simulink model "MulticopterModel"  (R2022a)
settings: Solver=ode4  StartTime=0.0  StopTime=inf  FixedStep=0.001  RelTol=1e-3
PreLoadFcn:
  | filepath  = fileparts(get_param(bdroot, 'FileName'));
  | cd(filepath);
InitFcn:
  | Init
values from neighbouring files (symbols this model uses):
  ModelFailEnable = 0    [Init.m]
  ModelInit_RPM = 0    [Init.m]
  ModelParam_BattHoverMinutes = 18    [Init.m]
  ModelParam_BattHoverThr = 0.609    [Init.m]
  ModelParam_envAltitude = -50    [Init.m]
  ModelParam_GlobalNoiseGainSwitch = 0.4    [Init.m]
  ModelParam_GPSEphFinal = 0.3    [Init.m]
  ModelParam_GPSEpvFinal = 0.4    [Init.m]
  ModelParam_GPSFix3DFix = 3    [Init.m]
  ModelParam_GPSSatsVisible = 10    [Init.m]
  ModelParam_motorCr = 842.1    [Init.m]
  ModelParam_motorJm = 0.0001287    [Init.m]
  ModelParam_motorMinThr = 0.05    [Init.m]
  ModelParam_motorT = 0.0214    [Init.m]
  ModelParam_motorWb = 22.83    [Init.m]
  ModelParam_noiseBaroCoupleWithSpeed = 0    [Init.m]
  ModelParam_noiseGPSSampTime = 0.2    [Init.m]
  ModelParam_noisePowerIMU = 0    [Init.m]
  ModelParam_noisePowerOffGainAccel = 0.04    [Init.m]
  ModelParam_noisePowerOffGainAccelZ = 0.03    [Init.m]
  ModelParam_noisePowerOffGainGyro = 0.02    [Init.m]
  ModelParam_noisePowerOffGainGyroZ = 0.025    [Init.m]
  ModelParam_noisePowerOffGainMag = 0.02    [Init.m]
  ModelParam_noisePowerOffGainMagZ = 0.035    [Init.m]
  ModelParam_noisePowerOnGainAccel = 0.8    [Init.m]
  ModelParam_noisePowerOnGainAccelZ = 4.5    [Init.m]
  ModelParam_noisePowerOnGainGyro = 2    [Init.m]
  ModelParam_noisePowerOnGainGyroZ = 1    [Init.m]
  ModelParam_noisePowerOnGainMag = 0.025    [Init.m]
  ModelParam_noisePowerOnGainMagZ = 0.05    [Init.m]
  ModelParam_noiseSampleTimeAccel = 0.001    [Init.m]
  ModelParam_noiseSampleTimeGyro = 0.001    [Init.m]
  ModelParam_noiseSampleTimeMag = 0.01    [Init.m]
  ModelParam_noiseUpperGPS = 0.5    [Init.m]
  ModelParam_noiseUpperWindBodyRatio = 0    [Init.m]
  ModelParam_noiseWindSampTime = 0.001    [Init.m]
  ModelParam_rotorCm = 2.783e-07    [Init.m]
  ModelParam_rotorCt = 1.681e-05    [Init.m]
  ModelParam_uavCCm = [0.0035 0.0039 0.0034]    [Init.m]
  ModelParam_uavCd = 0.055    [Init.m]
  ModelParam_uavDearo = 0.12    [Init.m]
  ModelParam_uavJ = [ModelParam_uavJxx,0,0;0,ModelParam_uavJyy,0;0,0,ModelParam_uavJzz]    [Init.m]
  ModelParam_uavMass = 1.515    [Init.m]
  ModelParam_uavMotNumbs = int8(4)    [Init.m]
  ModelParam_uavR = 0.225    [Init.m]
  ModelParam_uavType = int8(3)    [Init.m]
undefined symbols (not defined in the file or in its folder): d_i, Earth, h_i, ModelParam_GPSEpvInitial, ModelParam_GPSEpvTimeConstant, ModelParam_noiseLowPassFilterCoeAccel, ModelParam_noiseLowPassFilterCoeGyro, ModelParam_timeSamp, Newton, Raphson, WGS84
libraries: simulink x12, aerolibtransform2 x3, sharedtransform x3, aerolibasang x3, aerolibatmos2 x2, aerolibutil x2, shared6dof x1, aerolibconvert2 x1, aerolibobsolete x1, MulticopterModelLib x1, aerolibnav x1, aerolibgravity2 x1
(part 3 of 3)

== matlab function MulticopterModel/Force and Moment Model/Propeller Model/Multicopter/uavTypeDefine ==
  data: uavType input; n_p output; motorPhiVector output; motorThetaVector output; motorPsiVector output; motorRotateDirectionVector output
function [n_p,motorPhiVector,motorThetaVector,motorPsiVector,motorRotateDirectionVector]  = fcn(uavType)
% -1: anticlockwise, 1: clockwise 
TypeMotorDirMatrix=[...
    [-1 -1 -1 0 0 0 0 0];... % Tri 3*1 X           Type1
    [1 1 1 0 0 0 0 0];...    % Tri 3*1 +            Type2
    [-1 -1 1 1 0 0 0 0];... % Quad 4*1 X        Type3
    [-1 -1 1 1 0 0 0 0];... % Quad 4*1 +        Type4
    [1 -1 1 -1 -1 1 0 0];... % Hex 6*1 X         Type5
    [1 -1 1 -1 -1 1 0 0];... % Hex 6*1 +         Type6
    [1 -1 1 -1 1 -1 0 0];... % HexCoa 3*2      Type7
    [1 1 -1 -1 -1 -1 1 1];... % Oct 8*1 X        Type8
    [1 1 -1 -1 -1 -1 1 1];... % Oct 8*1 +        Type9
    [1 -1 1 -1 1 -1 1 -1];... % OctCoa 4*2 X  Type10
    [-1 -1 1 1 0 0 0 0];... % Intel Aero          Type11
    [-1 -1 1 1 0 0 0 0];... % custom              Type12
];

TypeMotorPsiAngMatrix=[...
    [pi/3 pi -pi/3 0 0 0 0 0];...%Type1
    [pi/3 pi -pi/3 0 0 0 0 0];...%Type2
    [pi/4   pi/4+pi     pi/4+3*pi/2     pi/4+pi/2   0 0 0 0];...%Type3
    [pi/2 3*pi/2 0 pi 0 0 0 0];...%Type4
    [pi/2 3/2*pi 3/2*pi+pi/3 pi/2+pi/3 pi/2-pi/3 3/2*pi-pi/3 0 0];...%Type5
    [0 pi pi+pi/3 pi/3 -pi/3 pi-pi/3 0 0];...%Type6
    [pi/3 pi/3 pi pi -pi/3 -pi/3 0 0];...%Type7
    [pi/8 pi+pi/8 pi/8+pi/4 pi-pi/8 -pi/8 3/2*pi-pi/8 3/2*pi+pi/8 pi/2+pi/8];...%Type8
    [0 pi pi/4 3/4*pi -pi/4 pi+pi/4 3/2*pi pi/2];...%Type9
    [pi/4 -pi/4 pi+pi/4 pi-pi/4 -pi/4 pi/4 pi-pi/4 pi+pi/4];...%Type10
    [43*pi/180     223*pi/180      317*pi/180      137*pi/180     0 0 0 0];...%Type11  Intel Aero
    [pi/4   pi/4+pi     pi/4+3*pi/2     pi/4+pi/2   0 0 0 0];...%Type12  custom
];

TypeMotorThetaAngMatrix=[...
    [0 0 0 0 0 0 0 0];...%Type1
    [0 0 0 0 0 0 0 0];...%Type2
    [0 0 0 0 0 0 0 0];...%Type3
    [0 0 0 0 0 0 0 0];...%Type4
    [0 0 0 0 0 0 0 0];...%Type5
    [0 0 0 0 0 0 0 0];...%Type6
    [0 0 0 0 0 0 0 0];...%Type7
    [0 0 0 0 0 0 0 0];...%Type8
    [0 0 0 0 0 0 0 0];...%Type9
    [0 0 0 0 0 0 0 0];...%Type10
    [0 0 0 0 0 0 0 0];...%Type11
    [pi/4   pi/4    pi/4    pi/4    0 0 0 0];...%Type12
    ];
TypeMotorPhiAngMatrix=[...
    [0 0 0 0 0 0 0 0];...%Type1
    [0 0 0 0 0 0 0 0];...%Type2
    [0 0 0 0 0 0 0 0];...%Type3
    [0 0 0 0 0 0 0 0];...%Type4
    [0 0 0 0 0 0 0 0];...%Type5
    [0 0 0 0 0 0 0 0];...%Type6
    [0 0 0 0 0 0 0 0];...%Type7
    [0 0 0 0 0 0 0 0];...%Type8
    [0 0 0 0 0 0 0 0];...%Type9
    [0 0 0 0 0 0 0 0];...%Type10
    [0 0 0 0 0 0 0 0];...%Type11
    [0 0 0 0 0 0 0 0];...%Type12
];

TypeMotorNonVector=int8([3;3;4;4;6;6;6;8;8;8;4;4]);

if uavType<0||uavType>length(TypeMotorNonVector)
    uavType=int8(1);
end

motorRotateDirectionVector=TypeMotorDirMatrix(uavType,:);
motorPsiVector=TypeMotorPsiAngMatrix(uavType,:);
motorThetaVector=TypeMotorThetaAngMatrix(uavType,:);
motorPhiVector=TypeMotorPhiAngMatrix(uavType,:);
n_p = TypeMotorNonVector(uavType);

== matlab function MulticopterModel/Force and Moment Model/Propeller Model/Car/MATLAB Function ==
  data: Fb output; Mb output; MotorRads input
function [Fb,Mb] = fcn(MotorRads)

Mb = [0;0;0];
Fb = [0;0;0];

Fb(1)=MotorRads(1)+MotorRads(3);
Mb(3)=MotorRads(1)*0.1-MotorRads(3)*0.1;

== matlab function MulticopterModel/OutputPort1/HILGPSModel/GenCogVel ==
  data: v output; u input; cot output
function [v,cot] = Ang360(u)
v=norm(u(1:2));

if v < 1
    cot = 0;
else
    cot=atan2d(u(2),u(1));
end
 
if cot<0
    cot=cot+360;
end

== matlab function MulticopterModel/Force and Moment Model/Body AeroCenter ==
  data: Fd output; Md output; wb input; Vb input; Cd input; CCm input; uavDearo input
function [Fd,Md] = fcn(wb,Vb,Cd, CCm, uavDearo)
% This is control effectiveness model, where Fb is the force produced by motors, Mb is
% the moment produced by motors, and Fd is the resistance produced by the air.
% The gyroscopic torque is not considered here.
% uavDearo 机身重心位置，向下为正

 Fd = -Cd*Vb.*abs(Vb);%
 
 Mfd=[Fd(2)*uavDearo;-Fd(1)*uavDearo;0];
 
Md=-CCm.*wb.*abs(wb);
Md=Mfd+Md;
%  CCm=4.72e-3;
%  Md=-CCm*wb.*abs(wb)*0.5;%0.3
%  Md= Mfd+Md;
 
end

== matlab function MulticopterModel/OutputPort1/Model Fail Assessment ==
  settings: updateMethod=DISCRETE
  data: ModelFailEnable input; landed input; FailInfo output; ve input; xe input; wb input; ang input
function FailInfo  = fcn(ModelFailEnable,landed,ve,xe,wb,ang)

persistent xTemp;
if isempty(xTemp)
     xTemp=zeros(8,1);
end

persistent kk;
if isempty(kk)
     kk=0;
end

persistent ss;
if isempty(ss)
     ss=zeros(6,1);
end

if ~ModelFailEnable&&(kk<0.5)
    xTemp=zeros(8,1);
    kk=0;
    ss=[xe;ang];
end

if ModelFailEnable&&~landed
    xTemp(1:4,1)=[norm(xe-ss(1:3,1));norm(ve);norm(ang-ss(4:6,1));norm(wb)];
    xTemp(5:8,1)= (xTemp(5:8,1)*kk+xTemp(1:4,1))/(kk+1);
    
    kk=kk+1;
end
%landed = int8(0);
 
FailInfo=xTemp;

== matlab function MulticopterModel/OutputPort1/ZLimit ==
  data: zt input; xe input; Xee output
function Xee = fcn(zt,xe)
Xee=xe;
if Xee(3)>zt
    Xee(3)=zt;
end

== matlab function MulticopterModel/CollisionDetection ==
  settings: updateMethod=DISCRETE
  data: fm output; uFloats input; DCM input; ve input; mass input; t input; tz output; isCrash output
function [fm,tz,isCrash] = fcn(uFloats,DCM,ve,mass,t)

% vect=[1;1;1;1;1;1;1;1];
%是否碰撞标志位
persistent isCol;
if isempty(isCol)
    isCol=int8(0);
end

%输出力和力矩暂存向量
persistent fOut;
if isempty(fOut)
    fOut=[0;0;0;0;0;0];
end    

%碰撞冲量矩阵
persistent mv0;
if isempty(mv0)
    mv0=[0;0;0];
end    

%碰撞时间
persistent tColi;
if isempty(tColi)
    tColi=0;
end      

%如果没有发送碰撞
if isCol<0.5
    %如果收到碰撞消息，且被碰撞物体为编号飞机（带CopterID的值大于0）
    if abs(uFloats(1)-12345)<1 && uFloats(2)>0.5 %如果收到碰撞消息，12345是数据校验位，uFloats(2)是碰撞到飞机的ID
        isCol=int8(1);%设置为碰撞模式
        %被碰撞物体是活动的还是固定的
        if uFloats(3)>0 %被碰撞物与本物体的质量比有正值，说明碰撞物也是飞机，需要用冲量定理
            massOb=mass*uFloats(3)^2;
            veOb = uFloats(7:9); 
            veNew=(mass*ve+massOb*veOb)/(mass+massOb);
        else %被碰撞物为树、房子等固定物体，质量无穷大，直接反弹回去（1/10的速度）
            veNew=-ve/10.0;
        end

        mv0=mass*(veNew-ve);
        tColi=t;%记录碰撞时间
    end        
end

%如果已经发生碰撞
if isCol>=0.5
    if (t-tColi)>0.05
        fOut=[0;0;0;0;0;0];
    else
        %用瞬时的作用力模拟冲量作用（0.05s）
        mv=DCM*mv0;
        mv(1)=mv(1)*(0.7+0.3*rand());
        mv(2)=mv(2)*(0.7+0.3*rand());
        mv(3)=mv(3)*(0.7+0.3*rand());
        fOut(1:3) = mv/0.05;    %冲量除以时间得到力
        fOut(4:6) = rand(3,1)*mass;
    end  
end

%下面处理飞机与场景固定物体之间的碰撞
fm = fOut;
%tz分别表示距地面高度和飞机XYZ坐标
tz=[100;0;0;0];
ddm=[0;0;0;0;0;0];  
if abs(uFloats(1)-12345)<1 %如果收到碰撞消息
    kRa=40;
    kRaVe=5;
    if uFloats(2)<0.5 %如果碰撞的是场景固定物体
        %向下照射射线返回长度
        tz(1)=uFloats(15);
        %飞机在UE4中的坐标
        tz(2:4)=uFloats(4:6);
    else        
        kRa=20;
    end  
    %前后左右是以地面坐标系的北东地为准
    %前障碍物碰撞反馈力
    if uFloats(10)<0 %距前墙面距离，小于0说明已经接触
        z=uFloats(10);
        if z>-0.01
            ddm(1)=-10*ve(1); 
        elseif z>-0.04
            ddm(1)=200*z-20*ve(1); 
        else
            ddm(1)=500*z-50*ve(1); 
        end   
    end
    %后障碍物碰撞反馈力
    if uFloats(11)<0
%         ddm(1)=-uFloats(11)*mass*kRa;
%         if ve(1)<0
%             ddm(1)=ddm(1)-ve(1)*mass*kRaVe;
%         end
        z=uFloats(11);
        if z>-0.01
            ddm(1)=-10*ve(1); 
        elseif z>-0.04
            ddm(1)=-200*z-20*ve(1); 
        else
            ddm(1)=-500*z-50*ve(1); 
        end  

    end 
    %左障碍物碰撞反馈力
    if uFloats(12)<0
%         ddm(2)=-uFloats(12)*mass*kRa;
%         if ve(2)<0
%             ddm(2)=ddm(2)-ve(2)*mass*kRaVe;
%         end
        z=uFloats(12);
        if z>-0.01
            ddm(2)=-10*ve(2); 
        elseif z>-0.04
            ddm(2)=-200*z-20*ve(2); 
        else
            ddm(2)=-500*z-50*ve(2); 
        end 
    end 
    %右障碍物碰撞反馈力
    if uFloats(13)<0
%         ddm(2)=uFloats(13)*mass*kRa;
%         if ve(2)>0
%             ddm(2)=ddm(2)-ve(2)*mass*kRaVe;
%         end
        z=uFloats(13);
        if z>-0.01
            ddm(2)=-10*ve(2); 
        elseif z>-0.04
            ddm(2)=200*z-20*ve(2); 
        else
            ddm(2)=500*z-50*ve(2); 
        end 

    end 
    %上障碍物碰撞反馈力
    if uFloats(14)<0
%         ddm(3)=-uFloats(14)*mass*kRa;
%         if ve(3)<0
%             ddm(3)=ddm(3)-ve(3)*mass*kRaVe;
%         end

        z=uFloats(14);
        if z>-0.01
            ddm(3)=-10*ve(3); 
        elseif z>-0.04
            ddm(3)=-200*z-20*ve(3); 
        else
            ddm(3)=-500*z-50*ve(3); 
        end 
    end
end
%力从地面坐标系映射机体坐标系
ddmm=DCM*ddm(1:3);
fm=fm+[ddmm;0;0;0];

isCrash=isCol;

== matlab function MulticopterModel/OutputPort1/HILGPSModel/MATLAB Function ==
  data: eph input; FixType output
function FixType = fcn(eph)
if eph <= 2
    FixType=3;
elseif eph <= 4
    FixType=2;
else
    FixType=0;
end

== matlab function MulticopterModel/MATLAB Function ==
  settings: updateMethod=DISCRETE
  data: TerrainZ input; y output; tz input
function y = fcn(TerrainZ, tz)
y=TerrainZ;
if tz(1)<=99
    y=tz(4)+tz(1);
end

% persistent last;
% if isempty(last)
%     last=TerrainZ;
% end
% y=TerrainZ;
% if tz(1)<10
%     if tz(1)<0
%         y=last;
%     else
%         y=tz(3)+tz(1);
%     end 
% end

== matlab function MulticopterModel/Crash_Motor_Fault ==
  settings: updateMethod=DISCRETE
  data: u input; y output; isCrash input
function y = fcn(u,isCrash)
y = u;



%如果飞机相撞则损坏三个电机
if isCrash>0.5
    y(1)=rand()/2.0;
    y(2)=rand()/5.0;
    y(3)=rand()/10.0+u(3)*0.9;
end

== matlab function MulticopterModel/Fail Model/Model Failure ==
  settings: updateMethod=DISCRETE
  data: T input; uavMass input; uavR input; isLoadFall input; uavlostMass output; uavlostJ output; LoadFallParams input; isLoadShift input; LoadShiftParams input; isLoadLeak input; LoadLeakParams input; dcm input; deltaM output
function [uavlostMass,uavlostJ,deltaM] = fcn(T,uavMass,uavR,isLoadFall,LoadFallParams,isLoadShift,LoadShiftParams,isLoadLeak,LoadLeakParams,dcm)
% This function aims to calculate the variation of mass and moment of
% inertia caused by model failure including LoadFall, LoadShift, and
% LoadLeak.

persistent tOld;
if isempty(tOld)  
   tOld=0;
end    

deltaM=[0;0;0];

if isLoadFall
    if LoadFallParams(1)>0.95
        LoadFallParams(1)=0.95;
    elseif LoadFallParams(1)<0
        LoadFallParams(1)=0;
    end
    uavlostMass=LoadFallParams(1)*uavMass;
    uavlostJ=zeros(3,3);
elseif isLoadShift
    if LoadShiftParams(1)>0.95
        LoadShiftParams(1)=0.95;
    elseif LoadShiftParams(1)<0
        LoadShiftParams(1)=0;
    end
    
    uavlostMass= 0;
    loadMoveMass= LoadShiftParams(1)*uavMass;
    
    X=uavR*LoadShiftParams(2);
    Y=uavR*LoadShiftParams(3);
    Z=uavR*LoadShiftParams(4);
    
    uavlostJxx= loadMoveMass*(Y^2+Z^2);
    uavlostJyy= loadMoveMass*(X^2+Z^2);
    uavlostJzz= loadMoveMass*(X^2+Y^2);
    uavlostJyz= loadMoveMass*Y*Z;
    uavlostJzx= loadMoveMass*Z*X;
    uavlostJxy= loadMoveMass*X*Y;
    uavlostJ=-[uavlostJxx,-uavlostJxy,-uavlostJzx;-uavlostJxy,uavlostJyy,-uavlostJyz;-uavlostJzx,-uavlostJyz,uavlostJzz];
    
    deltaF = dcm*loadMoveMass*[0;0;9.8];
    
    deltaM = cross([X;Y;Z],deltaF);     % 变化的力矩
    
elseif isLoadLeak
    uavlostJ=zeros(3,3);
    if LoadLeakParams(1)>0.99
        LoadLeakParams(1)=0.99;
    elseif LoadLeakParams(1)<0
        LoadLeakParams(1)=0;
    end
    loadmass0=LoadLeakParams(1)*uavMass;
    
    if tOld<0.01
        tOld=T;
    end
    
    dt=T-tOld;
    
    LoadLeakRatio = LoadLeakParams(2)*dt;
    if LoadLeakRatio > 0.99
        LoadLeakRatio = 0.99;
    end
    uavlostMass = LoadLeakRatio*loadmass0;
    
else
    uavlostMass=0;
    uavlostJ=zeros(3,3);
    tOld=0;
end

if ~isLoadLeak    %reset
    tOld=0;
end

== matlab function MulticopterModel/Force and Moment Model/Propeller Model old Version ==
  data: uavType input; MotorRads input; R input; uavDearo input; Fb output; Mb output; Cm input; Ct input; Jm input; wb input; Vb input; Cd input
function [Fb,Mb] = fcn(uavType,MotorRads,R,uavDearo,Cm,Ct,Jm,wb,Vb,Cd)
% This is control effectiveness model, where Fb is the force produced by motors, Mb is
% the moment produced by motors, and Fd is the resistance produced by the air.
% The gyroscopic torque is not considered here.

% -1: anticlockwise, 1: clockwise 
TypeMotorDirMatrix=[...
    [-1 -1 -1 0 0 0 0 0];... % Tri 3*1 X
    [1 1 1 0 0 0 0 0];...    % Tri 3*1 +
    [-1 -1 1 1 0 0 0 0];... % Quad 4*1 X
    [-1 -1 1 1 0 0 0 0];... % Quad 4*1 +
    [1 -1 1 -1 -1 1 0 0];... % Hex 6*1 X
    [1 -1 1 -1 -1 1 0 0];... % Hex 6*1 +
    [1 -1 1 -1 1 -1 0 0];... % HexCoa 3*2
    [1 1 -1 -1 -1 -1 1 1];... % Oct 8*1 X
    [1 1 -1 -1 -1 -1 1 1];... % Oct 8*1 +
    [1 -1 1 -1 1 -1 1 -1];... % OctCoa 4*2 X
];

TypeMotorAngMatrix=[...
    [pi/3 pi -pi/3 0 0 0 0 0];...
    [pi/3 pi -pi/3 0 0 0 0 0];...
    [pi/4 pi/4+pi pi/4+3*pi/2 pi/4+pi/2 0 0 0 0];...
    [pi/2 3*pi/2 0 pi 0 0 0 0];...
    [pi/2 3/2*pi 3/2*pi+pi/3 pi/2+pi/3 pi/2-pi/3 3/2*pi-pi/3 0 0];...
    [0 pi pi+pi/3 pi/3 -pi/3 pi-pi/3 0 0];...
    [pi/3 pi/3 pi pi -pi/3 -pi/3 0 0];...
    [pi/8 pi+pi/8 pi/8+pi/4 pi-pi/8 -pi/8 3/2*pi-pi/8 3/2*pi+pi/8 pi/2+pi/8];...
    [0 pi pi/4 3/4*pi -pi/4 pi+pi/4 3/2*pi pi/2];...
    [pi/4 -pi/4 pi+pi/4 pi-pi/4 -pi/4 pi/4 pi-pi/4 pi+pi/4];...
];

TypeMotorNonVector=int8([3;3;4;4;6;6;6;8;8;8]);

Mb = [0;0;0];
Fb = [0;0;0];
P=wb(1);Q=wb(2);

if uavType==50
    
    Fb(1)=MotorRads(1)+MotorRads(3);
    Mb(3)=MotorRads(1)*0.1-MotorRads(3)*0.1;
    
    return;
end


if uavType<0||uavType>length(TypeMotorNonVector)
    uavType=int8(1);
end

TypeMotorDirVector=TypeMotorDirMatrix(uavType,:);
TypeMotorAngVector=TypeMotorAngMatrix(uavType,:);

for i=1:TypeMotorNonVector(uavType)
    propAng = TypeMotorAngVector(i);
    propdir = TypeMotorDirVector(i);
    PropT = Ct*MotorRads(i)*MotorRads(i);
    PropM = Cm*MotorRads(i)*MotorRads(i);
    
    %Thrust -> Moment
    Mb=Mb+[-R*sin(propAng)*PropT;R*cos(propAng)*PropT;-PropM*propdir];
    
    %gyroscopic moment
    Mb=Mb+[Q*Jm*MotorRads(i)*propdir;-P*Jm*MotorRads(i)*propdir;0];
    
    Fb=Fb+[0;0;-PropT];
end

 
end

== matlab function MulticopterModel/Force and Moment Model/Ground Model ==
  settings: updateMethod=DISCRETE
  data: mg input; wb input; Xe input; F1 output; Ve input; M1 output; Quet input; terrainZ input; landed output; takeoff output
function [F1,M1,landed,takeoff] = fcn(mg,wb,Xe,Ve,Quet,terrainZ)
% This is a ground model that can provides reaction force and reaction torque

% persistent z0;
% if isempty(z0)
%      z0=0;
% end

persistent takeoffFlag;
if isempty(takeoffFlag)
     takeoffFlag=int8(0);
end

persistent landFlag;
if isempty(landFlag)
     landFlag=int8(1);
end

z=Xe(3)-terrainZ;

if (z<-0.3)&&(Ve(3)<-0.1)&&(takeoffFlag<0.5)
    takeoffFlag=int8(1);
    landFlag=int8(0);
end

if (z>-0.05)&&(Ve(3)>0.1)&&(landFlag<0.5)
    landFlag=int8(1);
    takeoffFlag=int8(0);
end

takeoff = takeoffFlag;
landed = landFlag;


F1=[0;0;0];
M1=[0;0;0];

if z>=0
%     if z>=0.3
%         if Ve(3)>=5
%             F1(3)=-mg(3)-1000*Ve(3);
%         else
%             F1(3)=-mg(3)-500*z-100*Ve(3);  
%         end
%     elseif z>=0.1
%         if Ve(3)>=2
%             F1(3)=-mg(3)-100*Ve(3);
%         else
%             F1(3)=-mg(3)-50*z-100*Ve(3);  
%         end
%     else
%          if Ve(3)>=1
%             F1(3)=-mg(3)-50*Ve(3);
%         else
%             F1(3)=-mg(3)-5*z-50*Ve(3);  
%         end       
%     end
    if z<0.05
        F1(3)=-mg(3)-10*Ve(3); 
    elseif z<0.1
        F1(3)=-mg(3)-0.5*z-20*Ve(3); 
    else
        F1(3)=-mg(3)-1*z-50*Ve(3); 
    end

    F1(1)=-50*Ve(1);
    F1(2)=-50*Ve(2);
    
%     if ~(isnan(Quet(2))||isnan(Quet(3))||isnan(Quet(4)))
%         M1=-200*[Quet(2);Quet(3);Quet(4)]-10*wb;
%     end
    
    M1=-20*[Quet(2);Quet(3);Quet(4)]-5*wb;
    M1 = M1 * abs(mg(3))*0.0333;
end

== matlab function MulticopterModel/Battery Model/MATLAB Function ==
  data: load input; time input; EffRatio output; hover_time input; hover_thr input; motorNumbs input; cell_voltage output; isUseCustomHovTime input; CustomHovTime input; isPowOff input; isLowVoltage input; remainVoltageRatio input; islowCapacity input; remainCapacityRatio input; remCapacity output
function [EffRatio, cell_voltage,remCapacity]= LiPo(load,time,hover_time,hover_thr,motorNumbs,isUseCustomHovTime,CustomHovTime,isPowOff,isLowVoltage,remainVoltageRatio,islowCapacity,remainCapacityRatio)
%% battery model
%================================Constants=================================

delta_t = 0.01;
%max_current = 5.500;                % maximum current per motor             (A)
%aux_current = 0.100;                % current of auxillary components       (A)        
%capacity = 1.000;                   % LiPo current capacity                 (Ah)                                 
%cells = 2;                          % LiPo cell count

%==========================================================================

persistent discharge;
if isempty(discharge)
    discharge = 0;
end

persistent startTime;
if isempty(startTime)
    startTime = 0;
end

persistent reset;
if isempty(reset)
    reset = 0;
end

discharge_capacity=0;

% 低电量故障
if islowCapacity
   hover_time = hover_time*remainCapacityRatio(1);
   isUseCustomHovTime=false;
end


if ~isUseCustomHovTime 
    capacity=1;
    
    if hover_time<0.01
        hover_time=0.01;
    end
    
    hover_current=1/(hover_time*1.4/60);
    current=0;
    for i=1:motorNumbs
        current=current+hover_current*(load(i)/hover_thr)^2;
    end
    aux_current=0.5;
    %current = sum(hover_current .* (load/hover_thr).^2) + aux_current;
    current =(current+aux_current)/double(motorNumbs);
    discharge = current * (delta_t / 3600) + discharge;
    discharge_capacity = discharge / capacity;    
end




%如果启用电池模型且使用自定义续航时间
if isUseCustomHovTime
      hover_time=CustomHovTime*1.4*60;
      if reset<0.5
         startTime=time;
         reset=1;
      end
      if hover_time<0.01
          hover_time=0.01;
      end
     discharge_capacity=(time-startTime)/hover_time;
else
    %使用默认的续航算法
    reset=0;
end


if discharge_capacity<0
    discharge_capacity=0;
end
if discharge_capacity>1
    discharge_capacity=1;
end


%电量与电压的曲线
if (0 <= discharge_capacity) && (discharge_capacity <=0.20)
    cell_voltage = -14.029*discharge_capacity^3 + 16.975*discharge_capacity^2 - 5.3339*discharge_capacity + 4.2;
elseif (0.20 < discharge_capacity) && (discharge_capacity < 0.70)
    cell_voltage = -0.2*discharge_capacity + 3.74;
else
    cell_voltage = -48*discharge_capacity^3 + 89.6*discharge_capacity^2 - 55.08*discharge_capacity + 14.716;
end

if cell_voltage < 0.5
    cell_voltage = 0;
end

% 电池失效故障
if isPowOff
     cell_voltage = 0; 
end

% 低电压故障
if isLowVoltage
    if remainVoltageRatio(1)>1
        remainVoltageRatio(1)=1;
    elseif remainVoltageRatio(1)<0
        remainVoltageRatio(1)=0;
    end
     cell_voltage = remainVoltageRatio(1)*4.2;
end


%如果电池模型未启用，续航为无穷久，同时各个全局变量归零
if ~isUseCustomHovTime&&~isPowOff&&~isLowVoltage&&~islowCapacity
    cell_voltage=4.2;
    discharge = 0;
    startTime = 0;
    reset = 0;
end

%效率矩阵
EffRatio=cell_voltage/4.2;
remCapacity=1-discharge_capacity;
%==========================================================================

== matlab function MulticopterModel/OutputPort1/HILGPSModel/-pi-pi---->0-2pi ==
  data: yaw180 input; yaw360 output
function yaw360 = fcn(yaw180)
%//rad
if yaw180>0
    yaw360 = yaw180;
else
    yaw360 = yaw180 +2*pi;
end
